simulink model "MainModel"  (R2023b)
settings: Solver=FixedStepAuto  StartTime=0.0  StopTime=20  FixedStep=0.001  MaxStep=0.01  RelTol=1e-3
values from neighbouring files (symbols this model uses):
  centers = linspace(center_range(1), center_range(2), num_nodes)    [main.m]    (also in main3.m)
  W = linspace(-1, 1, num_nodes)    [main.m]    (also in main3.m)
settings Model: Creator=Arshia  LastModifiedBy=GreenTeam

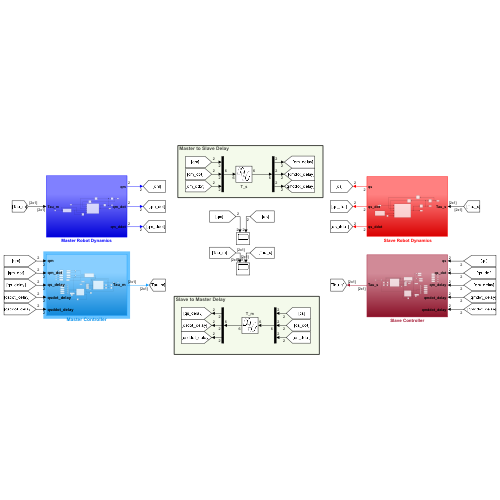
[thumbnail: Simulink's stored preview of the top-level diagram]
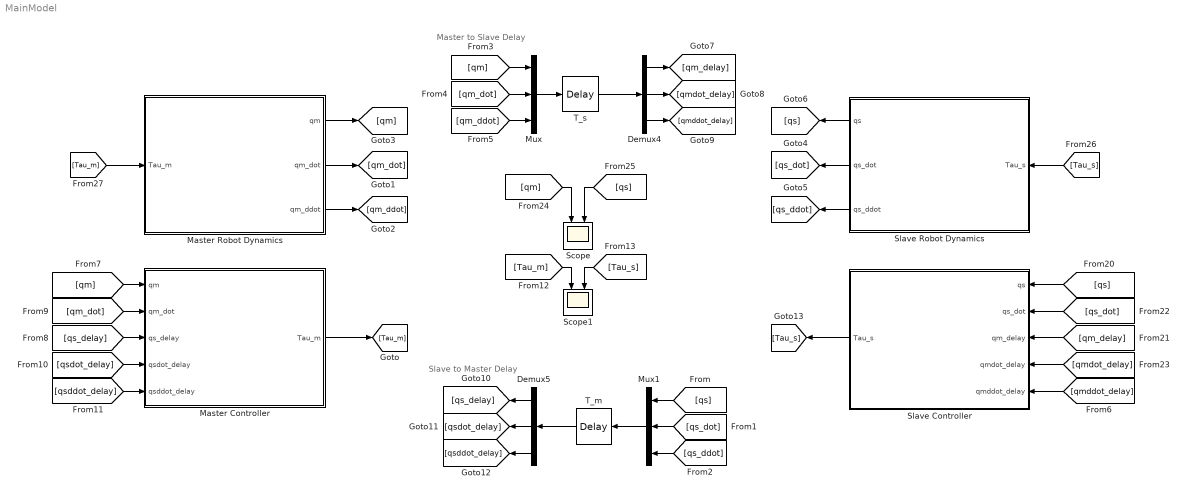
== system MainModel ==
  note: Master to Slave Delay
  note: Slave to Master Delay
  " Slave Robot Dynamics" : Subsystem
  Demux4 : Demux  Outputs=3
  Demux5 : Demux  Outputs=3
  Master Controller : Subsystem
  Master Robot Dynamics : Subsystem
  Mux : Mux  Inputs=3
  Mux1 : Mux  Inputs=3
  Scope : Scope  NumInputPorts=2
  Scope1 : Scope  NumInputPorts=2
  Slave Controller : Subsystem
      settings: PortSchema="{\"entries\":[{\"content\":{\"sides\":[{\"content\":{\"connectorIds\":[\"Out1\"]},\"type\":\"ConnectorPlacement.EquallySpacedRectSide\",\"uuid\":\"d4a5ddb8-0a78-4a6a-b69d-d0fbf887851f\"},{\"content\":{\"connectorIds\":[\"In1\",\"In2\",\"In3\",\"In4\",\"In5\"],\"side\":\"RIGHT\"},\"type\":\"ConnectorPlacement.EquallySpacedRectSide\",\"uuid\":\"c5c29000-cc93-4062-8d85-ef113d846d4c\"},{\"content\":{\"side\":\"TOP\"},\"type\":\"ConnectorPlacement.EquallySpacedRectSide\",\"uuid\":\"9fcdc3c0-dbe1-4ddf-bcf2-0add46548f02\"}]},\"type\":\"ConnectorPlacement.EquallySpacedConnector\",\"uuid\":\"1cc86ea2-f14f-4381-9537-68d258fe8551\"}],\"packageUris\":[\"http://schema.mathworks.com/mf0/Connector/R2020b\"],\"version\":\"1.0\"}"
  T_m : TransportDelay  DelayTime=0.6  BufferSize=1024*1024
  T_s : TransportDelay  DelayTime=0.6  BufferSize=1024*1024
  wires:
  Mux/1 -> T_s/1
  Mux1/1 -> T_m/1
  Master Robot Dynamics/1(qm) -> [qm]
  Master Robot Dynamics/2(qm_dot) -> [qm_dot]
  Master Robot Dynamics/3(qm_ddot) -> [qm_ddot]
  " Slave Robot Dynamics"/1(qs) -> [qs]
  " Slave Robot Dynamics"/3(qs_ddot) -> [qs_ddot]
  " Slave Robot Dynamics"/2(qs_dot) -> [qs_dot]
  [qs] -> Mux1/1
  [qs_dot] -> Mux1/2
  [qs_ddot] -> Mux1/3
  [qm] -> Mux/1
  [qm_dot] -> Mux/2
  [qm_ddot] -> Mux/3
  Demux4/1 -> [qm_delay]
  Demux4/2 -> [qmdot_delay]
  Demux4/3 -> [qmddot_delay]
  Demux5/1 -> [qs_delay]
  Demux5/3 -> [qsddot_delay]
  Demux5/2 -> [qsdot_delay]
  [qs] -> Scope/2
  [Tau_s] -> " Slave Robot Dynamics"/1(Tau_s)
  [Tau_m] -> Master Robot Dynamics/1(Tau_m)
  Master Controller/1(Tau_m) -> [Tau_m]
  Slave Controller/1(Tau_s) -> [Tau_s]
  [qs] -> Slave Controller/1(qs)
  [qm_delay] -> Slave Controller/3(qm_delay)
  [qs_dot] -> Slave Controller/2(qs_dot)
  [qmdot_delay] -> Slave Controller/4(qmdot_delay)
  [qmddot_delay] -> Slave Controller/5(qmddot_delay)
  [qm] -> Master Controller/1(qm)
  [qm_dot] -> Master Controller/2(qm_dot)
  [qs_delay] -> Master Controller/3(qs_delay)
  [qsdot_delay] -> Master Controller/4(qsdot_delay)
  [qsddot_delay] -> Master Controller/5(qsddot_delay)
  [Tau_s] -> Scope1/2
  [Tau_m] -> Scope1/1
  [qm] -> Scope/1
  T_m/1 -> Demux5/1
  T_s/1 -> Demux4/1

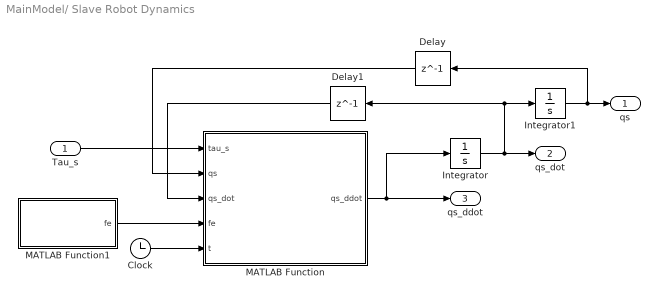
== system MainModel/ Slave Robot Dynamics ==
  Tau_s : Inport
  Clock : Clock
  Delay : Delay  DelayLength=1
  Delay1 : Delay  DelayLength=1
  Integrator : Integrator  InitialCondition=[0;0]
  Integrator1 : Integrator  InitialCondition=[0.25*pi; 0.1*pi]
  MATLAB Function : MATLAB Function  TreatAsAtomicUnit=on
  MATLAB Function1 : MATLAB Function  TreatAsAtomicUnit=on
  qs : Outport
  qs_dot : Outport  Port=2
  qs_ddot : Outport  Port=3
  wires:
  Clock/1 -> MATLAB Function/5(t)
  Integrator1/1 -> Delay/1, qs/1
  Integrator/1 -> Delay1/1, Integrator1/1, qs_dot/1
  MATLAB Function/1(qs_ddot) -> qs_ddot/1, Integrator/1
  Tau_s/1 -> MATLAB Function/1(tau_s)
  MATLAB Function1/1(fe) -> MATLAB Function/4(fe)
  Delay/1 -> MATLAB Function/2(qs)
  Delay1/1 -> MATLAB Function/3(qs_dot)

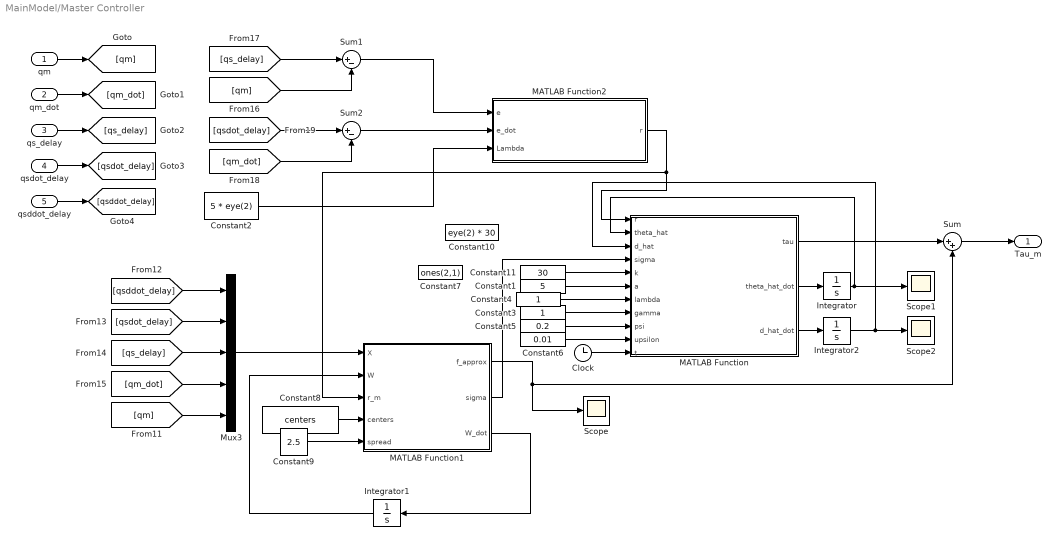
== system MainModel/Master Controller ==
  qm : Inport
  qm_dot : Inport  Port=2
  qs_delay : Inport  Port=3
  qsdot_delay : Inport  Port=4
  qsddot_delay : Inport  Port=5
  Clock : Clock
  Constant1 : Constant  Value=5
  Constant10 : Constant  Value=eye(2) * 30
  Constant11 : Constant  Value=30
  Constant2 : Constant  Value=5 * eye(2)
  Constant3 : Constant
  Constant4 : Constant
  Constant5 : Constant  Value=0.2
  Constant6 : Constant  Value=0.01
  Constant7 : Constant  Value=ones(2,1)
  Constant8 : Constant  Value=centers
  Constant9 : Constant  Value=2.5
  Integrator : Integrator  InitialCondition=[0;0]
  Integrator1 : Integrator  InitialCondition=W' .* eye(size(centers,1),2)
  Integrator2 : Integrator  InitialCondition=[0;0]
  MATLAB Function : MATLAB Function  TreatAsAtomicUnit=on
  MATLAB Function1 : MATLAB Function  TreatAsAtomicUnit=on
  MATLAB Function2 : MATLAB Function  TreatAsAtomicUnit=on
  Mux3 : Mux  Inputs=5
  Scope : Scope
  Scope1 : Scope
  Scope2 : Scope
  Sum : Sum  Inputs=|++
  Sum1 : Sum  Inputs=|+-
  Sum2 : Sum  Inputs=|+-
  Tau_m : Outport
  wires:
  Integrator1/1 -> MATLAB Function1/2(W)
  Constant4/1 -> MATLAB Function/7(lambda)
  Constant1/1 -> MATLAB Function/6(a)
  Integrator2/1 -> MATLAB Function/3(d_hat), Scope2/1
  Constant8/1 -> MATLAB Function1/4(centers)
  [qm] -> Sum1/2
  MATLAB Function/2(theta_hat_dot) -> Integrator/1
  [qm_dot] -> Mux3/4
  MATLAB Function/3(d_hat_dot) -> Integrator2/1
  MATLAB Function2/1(r) -> MATLAB Function1/3(r_m), MATLAB Function/1(r)
  Constant2/1 -> MATLAB Function2/3(Lambda)
  Constant6/1 -> MATLAB Function/10(upsilon)
  Constant5/1 -> MATLAB Function/9(psi)
  Mux3/1 -> MATLAB Function1/1(X)
  MATLAB Function1/2(sigma) -> MATLAB Function/4(sigma)
  Constant9/1 -> MATLAB Function1/5(spread)
  [qsddot_delay] -> Mux3/1
  [qsdot_delay] -> Sum2/1
  Constant11/1 -> MATLAB Function/5(k)
  Integrator/1 -> MATLAB Function/2(theta_hat), Scope1/1
  Clock/1 -> MATLAB Function/11(t)
  Constant3/1 -> MATLAB Function/8(gamma)
  Sum/1 -> Tau_m/1
  [qm_dot] -> Sum2/2
  [qm] -> Mux3/5
  Sum1/1 -> MATLAB Function2/1(e)
  [qs_delay] -> Sum1/1
  [qs_delay] -> Mux3/3
  [qsdot_delay] -> Mux3/2
  qs_delay/1 -> [qs_delay]
  qm/1 -> [qm]
  qm_dot/1 -> [qm_dot]
  qsdot_delay/1 -> [qsdot_delay]
  qsddot_delay/1 -> [qsddot_delay]
  Sum2/1 -> MATLAB Function2/2(e_dot)
  MATLAB Function1/3(W_dot) -> Integrator1/1
  MATLAB Function/1(tau) -> Sum/1
  MATLAB Function1/1(f_approx) -> Scope/1, Sum/2

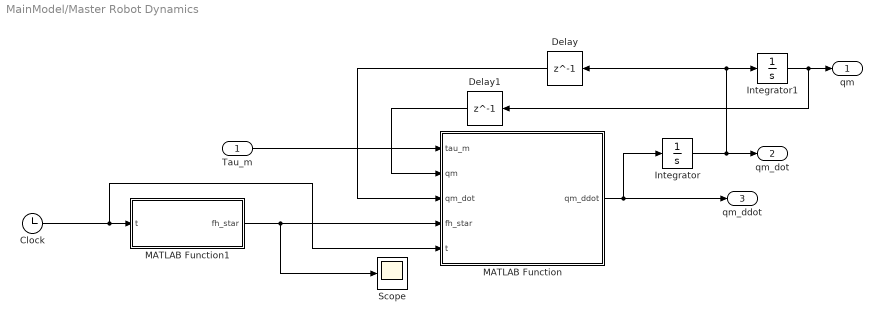
== system MainModel/Master Robot Dynamics ==
  Tau_m : Inport
  Clock : Clock
  Delay : Delay  DelayLength=1
  Delay1 : Delay  DelayLength=1
  Integrator : Integrator  InitialCondition=[0;0]
  Integrator1 : Integrator  InitialCondition=[0.4*pi; 0.2*pi]
  MATLAB Function : MATLAB Function  TreatAsAtomicUnit=on
  MATLAB Function1 : MATLAB Function  TreatAsAtomicUnit=on
  Scope : Scope
  qm : Outport
  qm_dot : Outport  Port=2
  qm_ddot : Outport  Port=3
  wires:
  Tau_m/1 -> MATLAB Function/1(tau_m)
  Clock/1 -> MATLAB Function/5(t), MATLAB Function1/1(t)
  MATLAB Function/1(qm_ddot) -> Integrator/1, qm_ddot/1
  Integrator/1 -> Integrator1/1, Delay/1, qm_dot/1
  Integrator1/1 -> Delay1/1, qm/1
  MATLAB Function1/1(fh_star) -> Scope/1, MATLAB Function/4(fh_star)
  Delay/1 -> MATLAB Function/3(qm_dot)
  Delay1/1 -> MATLAB Function/2(qm)

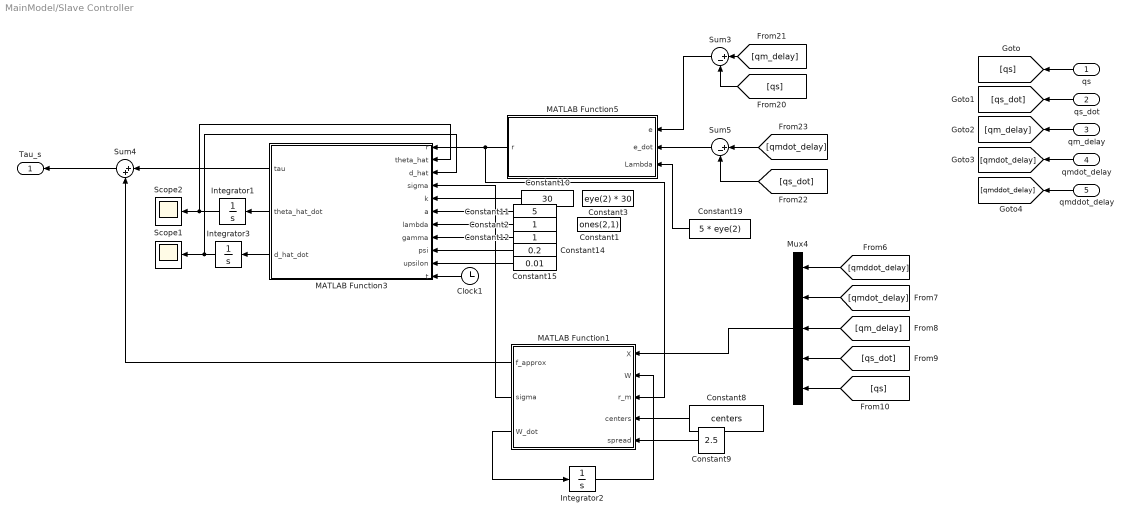
== system MainModel/Slave Controller ==
  qs : Inport
  qs_dot : Inport  Port=2
  qm_delay : Inport  Port=3
  qmdot_delay : Inport  Port=4
  qmddot_delay : Inport  Port=5
  Clock1 : Clock
  Constant1 : Constant  Value=ones(2,1)
  Constant10 : Constant  Value=30
  Constant11 : Constant  Value=5
  Constant12 : Constant
  Constant14 : Constant  Value=0.2
  Constant15 : Constant  Value=0.01
  Constant19 : Constant  Value=5 * eye(2)
  Constant2 : Constant
  Constant3 : Constant  Value=eye(2) * 30
  Constant8 : Constant  Value=centers
  Constant9 : Constant  Value=2.5
  Integrator1 : Integrator  InitialCondition=[0;0]
  Integrator2 : Integrator  InitialCondition=W' .* eye(size(centers,1),2)
  Integrator3 : Integrator  InitialCondition=[0;0]
  MATLAB Function1 : MATLAB Function  TreatAsAtomicUnit=on
  MATLAB Function3 : MATLAB Function  TreatAsAtomicUnit=on
  MATLAB Function5 : MATLAB Function  TreatAsAtomicUnit=on
  Mux4 : Mux  Inputs=5
  Scope1 : Scope
  Scope2 : Scope
  Sum3 : Sum  Inputs=|+-
  Sum4 : Sum  Inputs=|++
  Sum5 : Sum  Inputs=|+-
  Tau_s : Outport
  wires:
  [qs] -> Mux4/5
  Constant12/1 -> MATLAB Function3/8(gamma)
  Sum4/1 -> Tau_s/1
  Constant2/1 -> MATLAB Function3/7(lambda)
  MATLAB Function3/1(tau) -> Sum4/1
  Constant15/1 -> MATLAB Function3/10(upsilon)
  Integrator3/1 -> Scope1/1, MATLAB Function3/3(d_hat)
  Constant14/1 -> MATLAB Function3/9(psi)
  Constant19/1 -> MATLAB Function5/3(Lambda)
  Sum3/1 -> MATLAB Function5/1(e)
  Integrator1/1 -> Scope2/1, MATLAB Function3/2(theta_hat)
  Constant11/1 -> MATLAB Function3/6(a)
  [qmdot_delay] -> Sum5/1
  Clock1/1 -> MATLAB Function3/11(t)
  [qmdot_delay] -> Mux4/2
  MATLAB Function3/2(theta_hat_dot) -> Integrator1/1
  [qmddot_delay] -> Mux4/1
  Constant10/1 -> MATLAB Function3/5(k)
  MATLAB Function3/3(d_hat_dot) -> Integrator3/1
  [qm_delay] -> Sum3/1
  [qm_delay] -> Mux4/3
  [qs] -> Sum3/2
  [qs_dot] -> Mux4/4
  [qs_dot] -> Sum5/2
  qs/1 -> [qs]
  qs_dot/1 -> [qs_dot]
  qm_delay/1 -> [qm_delay]
  qmdot_delay/1 -> [qmdot_delay]
  qmddot_delay/1 -> [qmddot_delay]
  Sum5/1 -> MATLAB Function5/2(e_dot)
  MATLAB Function1/3(W_dot) -> Integrator2/1
  Constant8/1 -> MATLAB Function1/4(centers)
  MATLAB Function1/2(sigma) -> MATLAB Function3/4(sigma)
  Integrator2/1 -> MATLAB Function1/2(W)
  MATLAB Function5/1(r) -> MATLAB Function1/3(r_m), MATLAB Function3/1(r)
  Constant9/1 -> MATLAB Function1/5(spread)
  Mux4/1 -> MATLAB Function1/1(X)
  MATLAB Function1/1(f_approx) -> Sum4/2

== matlab function MainModel/Slave Controller/MATLAB Function1 ==
  data: X input; f_approx output; W input; r_m input; centers input; spread input; sigma output; W_dot output
function [f_approx, sigma, W_dot] = rbf_network(X, W, r_m, centers, spread)
% -------------------------------------------------------------------------
% RBF network and adaptive weight update (Eq. 44 of the paper)
%
% Inputs:
%   X        : input vector (state/regressor)
%   W        : current weight matrix (n_neurons × n_outputs)
%   r_m      : sliding variable vector (n_outputs × 1)
%   centers  : RBF centers (n_neurons × dim(X))
%   spread   : RBF width (scalar)
%
% Outputs:
%   f_approx : RBF network output  (n_outputs × 1)
%   sigma    : RBF activation vector (n_neurons × 1)
%   W_dot    : time derivative of weights (n_neurons × n_outputs)
% -------------------------------------------------------------------------

    %% --- Compute Gaussian basis functions (σ) ---
    n_neurons = size(centers,1);
    sigma = zeros(n_neurons,1);
    for i = 1:n_neurons
        sigma(i) = exp(-norm(X - centers(i,:))^2 / (spread^2));
    end

    %% --- Network output approximation ---
    % f ≈ Wᵀ σ
    f_approx = W' * sigma;   % (n_outputs×1)

    %% --- Adaptive law for weight update (Eq. 44) ---
    %   W_dot = Γ * σ * rᵀ - Γ * ψ * W
    Gamma = 1.0 * eye(n_neurons);     % adaptation gain (tune >0)
    psi   = 0.01;                     % small leakage term (0.001–0.05)

    % Weight derivative (each neuron adapts based on σ * rᵀ)
    W_dot = Gamma * (sigma * r_m') - Gamma * psi * W;
end

== matlab function MainModel/Slave Controller/MATLAB Function5 ==
  data: e input; r output; e_dot input; Lambda input
function r  = sliding_mode(e, e_dot, Lambda)
    r = e_dot + Lambda * e;
end

== matlab function MainModel/Master Robot Dynamics/MATLAB Function1 ==
  data: t input; fh_star output
function fh_star  = operator_force(t)
    % --- Desired operator force f_h*(t) (from paper) ---
    fh_star = [25*(1 - cos(0.5*pi*t)); 0];
end

== matlab function MainModel/Master Robot Dynamics/MATLAB Function ==
  data: tau_m input; qm_ddot output size=2; qm input; qm_dot input size=2; fh_star input; t input
function qm_ddot = master_dynamics(tau_m, qm, qm_dot, fh_star, t)
% -------------------------------------------------------------------------
% Master manipulator dynamics including operator hand dynamics
% (Implements Eqs. (9)-(11) of the paper)
%
% Inputs:
%   tau_m   : control torque (2×1)
%   qm      : joint positions (2×1)
%   qm_dot  : joint velocities (2×1)
%   fh_star : desired operator hand force f_h*(t) (2×1)
%   t       : current simulation time
%
% Output:
%   qm_ddot : joint accelerations (2×1)
% -------------------------------------------------------------------------

    %% --- Robot parameters (Table 2) ---
    mm1 = 0.5; lm1 = 0.6;
    mm2 = 0.5; lm2 = 0.4;
    g = 9.81;

    %% --- Human hand parameters (Table 2) ---
    Mh = 0.2;     % mass
    Bh = 50;      % damping
    Kh = 1000;    % stiffness

    %% --- Robot inertia (M_qm) ---
    q1 = qm(1); q2 = qm(2);
    q1_dot = qm_dot(1); q2_dot = qm_dot(2);

    M11 = mm1*lm1^2 + mm2*(lm1^2 + lm2^2 + 2*lm1*lm2*cos(q2));
    M12 = mm2*(lm2^2 + lm1*lm2*cos(q2));
    M21 = M12;
    M22 = mm2*lm2^2;
    M_qm = [M11 M12; M21 M22];

    %% --- Robot Coriolis (C_qm) ---
    C11 = -mm2*lm1*lm2*q2_dot*cos(q2);
    C12 = -mm2*lm1*lm2*(q1_dot + q2_dot)*sin(q2);
    C21 = mm2*lm1*lm2*q1_dot*sin(q2);
    C22 = 0;
    C_qm = [C11 C12; C21 C22];

    %% --- Robot gravity (G_qm) ---
    G1 = (mm1*lm2 + mm2*lm1)*g*cos(q1) + mm2*lm2*g*cos(q1 + q2);
    G2 = mm2*lm2*g*cos(q1 + q2);
    G_qm = [G1; G2];

    %% --- Jacobian and its derivative ---
    J = [ -lm1*sin(q1)-lm2*sin(q1+q2),  -lm2*sin(q1+q2);
           lm1*cos(q1)+lm2*cos(q1+q2),   lm2*cos(q1+q2) ];
    J_dot = [ -lm1*q1_dot*cos(q1) - lm2*(q1_dot+q2_dot)*cos(q1+q2),  -lm2*(q1_dot+q2_dot)*cos(q1+q2);
              -lm1*q1_dot*sin(q1) - lm2*(q1_dot+q2_dot)*sin(q1+q2),  -lm2*(q1_dot+q2_dot)*sin(q1+q2) ];

    %% --- End-effector position h(qm) ---
    hq = [lm1*cos(q1) + lm2*cos(q1+q2);
          lm1*sin(q1) + lm2*sin(q1+q2)];

    %% --- Augmented dynamics (Eqs. 9-11) ---
    M_m = M_qm + J' * Mh * J;
    C_m = C_qm + J' * Bh * J + J' * Mh * J_dot;
    G_m = G_qm + J' * Kh * hq - J' * fh_star;

    %% --- External disturbance (same form as before) ---
    f = [0.1*qm(1)*qm_dot(1)*sin(t);
         0.1*qm(2)*qm_dot(2)*sin(t)];

    %% --- Internal friction (Coulomb + viscous) ---
    fc = [qm_dot(1) + 3*sign(qm_dot(1));
          2*qm_dot(2) + 2*sign(qm_dot(2))];

    %% --- Solve for acceleration ---
    % According to Eq. (8): M_m*q̈m + C_m*q̇m + G_m = τ_m + Jᵀ f_h* - f - f_c
    %qm_ddot = pinv(M_m) * (tau_m - C_m*qm_dot - G_m - f - fc);
    qm_ddot = M_m \ (tau_m - C_m*qm_dot - G_m - f - fc);

end

== matlab function MainModel/ Slave Robot Dynamics/MATLAB Function ==
  data: tau_s input; qs input; qs_dot input size=2; fe input; t input; qs_ddot output size=2
function qs_ddot = slave_dynamics(tau_s, qs, qs_dot, fe, t)
% -------------------------------------------------------------------------
% Slave manipulator dynamics including environment interaction
% Implements Eqs. (8), (12), (13), (14) of the paper.
%
% Inputs:
%   tau_s   : control torque (2×1)
%   fe      : environment force (2×1)
%   qs      : joint positions (2×1)
%   qs_dot  : joint velocities (2×1)
%   t       : current simulation time
%
% Output:
%   qs_ddot : joint accelerations (2×1)
% -------------------------------------------------------------------------

    %% --- Robot parameters (Table 2) ---
    ms1 = 0.5; ls1 = 0.6;
    ms2 = 0.5; ls2 = 0.4;
    g = 9.81;

    %% --- Environment parameters (Table 2) ---
    Me = 0.1;    % environment mass
    Be = 20;     % environment damping
    Ke = 1000;   % environment stiffness

    %% --- Joint variables ---
    q1 = qs(1); q2 = qs(2);
    q1_dot = qs_dot(1); q2_dot = qs_dot(2);

    %% --- Robot inertia (M_qs) ---
    M11 = ms1*ls1^2 + ms2*(ls1^2 + ls2^2 + 2*ls1*ls2*cos(q2));
    M12 = ms2*(ls2^2 + ls1*ls2*cos(q2));
    M21 = M12;
    M22 = ms2*ls2^2;
    M_qs = [M11 M12; M21 M22];

    %% --- Robot Coriolis (C_qs) ---
    C11 = -ms2*ls1*ls2*q2_dot*cos(q2);
    C12 = -ms2*ls1*ls2*(q1_dot + q2_dot)*sin(q2);
    C21 =  ms2*ls1*ls2*q1_dot*sin(q2);
    C22 = 0;
    C_qs = [C11 C12; C21 C22];

    %% --- Robot gravity (G_qs) ---
    G1 = (ms1*ls2 + ms2*ls1)*g*cos(q1) + ms2*ls2*g*cos(q1 + q2);
    G2 = ms2*ls2*g*cos(q1 + q2);
    G_qs = [G1; G2];

    %% --- Jacobian and its derivative ---
    J = [ -ls1*sin(q1)-ls2*sin(q1+q2),  -ls2*sin(q1+q2);
           ls1*cos(q1)+ls2*cos(q1+q2),   ls2*cos(q1+q2) ];
    J_dot = [ -ls1*q1_dot*cos(q1) - ls2*(q1_dot+q2_dot)*cos(q1+q2),  -ls2*(q1_dot+q2_dot)*cos(q1+q2);
              -ls1*q1_dot*sin(q1) - ls2*(q1_dot+q2_dot)*sin(q1+q2),  -ls2*(q1_dot+q2_dot)*sin(q1+q2) ];

    %% --- End-effector position h(qs) ---
    hq = [ls1*cos(q1) + ls2*cos(q1+q2);
          ls1*sin(q1) + ls2*sin(q1+q2)];

    %% --- Augmented environment-coupled dynamics (Eqs. 12–14) ---
    M_s = M_qs + J' * Me * J;
    C_s = C_qs + J' * Be * J + J' * Me * J_dot;
    G_s = G_qs + J' * Ke * hq + J' * fe;

    %% --- External disturbance (optional; can remove for clean simulation) ---
    f = [0.1*qs(1)*qs_dot(1)*sin(t);
         0.1*qs(2)*qs_dot(2)*sin(t)];

    %% --- Internal friction (Coulomb + viscous, optional) ---
    fc = [3*qs_dot(1) + 4*sign(qs_dot(1));
          3*qs_dot(2) + 6*sign(qs_dot(2))];

    %% --- Solve for joint accelerations (Eq. 8) ---
    % M_s * q̈s + C_s * q̇s + G_s = τ_s - f - f_c
    qs_ddot = M_s \ (tau_s - C_s*qs_dot - G_s - f - fc);

end

== matlab function MainModel/ Slave Robot Dynamics/MATLAB Function1 ==
  data: fe output
function fe  = environment_force()
    fe = [0; 0];
end

== matlab function MainModel/Master Controller/MATLAB Function ==
  data: r input; tau output; theta_hat input; d_hat input; sigma input; k input; a input; lambda input; gamma input; psi input; upsilon input; theta_hat_dot output; d_hat_dot output; t input
function [tau, theta_hat_dot, d_hat_dot] = adaptive_controller(r, theta_hat, d_hat, sigma, k, a, lambda, gamma, psi, upsilon,t)
    % Control law (Equation 41)
    tau = k * r  + (r / (2 * a^2)) .* theta_hat * (sigma' * sigma) + (r / (norm(r) + exp(-a*t))) .* d_hat;
    % tau = k * r + (r / (norm(r) + eps)) .* f_approx + (r / (norm(r) + exp(-a*t))) .* d_hat;

    
    % Adaptive laws (Equations 44-45)
    theta_hat_dot = (lambda / (2 * a^2)) * (r' * r) * (sigma' * sigma) - psi * theta_hat;
    d_hat_dot = (gamma * (r' * r)) / (norm(r) + exp(-a*t)) - upsilon * d_hat;
end

== matlab function MainModel/Master Controller/MATLAB Function1 ==
  data: X input; f_approx output; W input; r_m input; centers input; spread input; sigma output; W_dot output
function [f_approx, sigma, W_dot] = rbf_network(X, W, r_m, centers, spread)
% -------------------------------------------------------------------------
% RBF network and adaptive weight update (Eq. 44 of the paper)
%
% Inputs:
%   X        : input vector (state/regressor)
%   W        : current weight matrix (n_neurons × n_outputs)
%   r_m      : sliding variable vector (n_outputs × 1)
%   centers  : RBF centers (n_neurons × dim(X))
%   spread   : RBF width (scalar)
%
% Outputs:
%   f_approx : RBF network output  (n_outputs × 1)
%   sigma    : RBF activation vector (n_neurons × 1)
%   W_dot    : time derivative of weights (n_neurons × n_outputs)
% -------------------------------------------------------------------------

    %% --- Compute Gaussian basis functions (σ) ---
    n_neurons = size(centers,1);
    sigma = zeros(n_neurons,1);
    for i = 1:n_neurons
        sigma(i) = exp(-norm(X - centers(i,:))^2 / (spread^2));
    end

    %% --- Network output approximation ---
    % f ≈ Wᵀ σ
    f_approx = W' * sigma;   % (n_outputs×1)

    %% --- Adaptive law for weight update (Eq. 44) ---
    %   W_dot = Γ * σ * rᵀ - Γ * ψ * W
    Gamma = 1.0 * eye(n_neurons);     % adaptation gain (tune >0)
    psi   = 0.01;                     % small leakage term (0.001–0.05)

    % Weight derivative (each neuron adapts based on σ * rᵀ)
    W_dot = Gamma * (sigma * r_m') - Gamma * psi * W;
end

== matlab function MainModel/Master Controller/MATLAB Function2 ==
  data: e input; r output; e_dot input; Lambda input
function r  = sliding_mode(e, e_dot, Lambda)
    r = e_dot + Lambda * e;
end

== matlab function MainModel/Slave Controller/MATLAB Function3 ==
  data: r input; tau output; theta_hat input; d_hat input; sigma input; k input; a input; lambda input; gamma input; psi input; upsilon input; theta_hat_dot output; d_hat_dot output; t input
function [tau, theta_hat_dot, d_hat_dot] = adaptive_controller(r, theta_hat, d_hat, sigma, k, a, lambda, gamma, psi, upsilon, t)
    % Control law (Equation 41)
    tau = k * r + (r ./ (2 * a^2)) .* theta_hat * (sigma' * sigma) + (r ./ (vecnorm(r) + exp(-a*t))) .* d_hat;
    %tau = k * r + (r / (norm(r) + eps)) .* f_approx + (r / (norm(r) + exp(-a*t))) .* d_hat;

    % Adaptive laws (Equations 44-45)
    theta_hat_dot = (lambda / (2 * a^2)) * (r' * r) * (sigma' * sigma) - psi * theta_hat;
    d_hat_dot = (gamma * (r' * r)) / (norm(r) + exp(-a*t)) - upsilon * d_hat;
end
